simulink library "M160_lib"  (Simulink 7.8)
settings: Solver=FixedStepDiscrete  StartTime=0.0  StopTime=10.0  RelTol=1e-3
PreLoadFcn:
  | update_path
undefined symbols (not defined in the file): Afr_atCool2facLambdaReqCorr_CUR_x, Afr_atCool2facLambdaReqCorr_CUR_y, Afr_atMani2facLambdaReqCorr_CUR_x, Afr_atMani2facLambdaReqCorr_CUR_y, Afr_facLambdaReqMan, Afr_facRatioMan, Afr_facStoich, Afr_flgLambdaReqOverride, Afr_flgRatioOverride, Afr_rpmEngSpdfacRelAir2facLambdaReqBase_MAP_x, Afr_rpmEngSpdfacRelAir2facLambdaReqBase_MAP_y, Afr_rpmEngSpdfacRelAir2facLambdaReqBase_MAP_z, Ais_flgAirInjReacPumpOverride, Ais_stAirInjReacPumpMan, Amc_flgAirMassFlowOverride, Amc_uSens2AirMassFlow_CUR_x, Amc_uSens2AirMassFlow_CUR_y, Amc_uSensMaxValid, Amc_uSensMinValid, Amf_facRelAirMan, Amf_flgAirMassPerStrOverride, Amf_flgRelAirOverride, Amf_flgSwitch2AirMassFlowMeter, Amf_mAirPerStrMan, Amf_pManiEngSpd2facRelAirCorr_MAP_x, Amf_pManiEngSpd2facRelAirCorr_MAP_y, Amf_pManiEngSpd2facRelAirCorr_MAP_z, Amf_rpmEngSpd2facTempCorr_CUR_x, Amf_rpmEngSpd2facTempCorr_CUR_y, Amf_shcSpecGasConst_C, Amf_volEngDisp_C, Apv_facAirPumpRateMan, Apv_factor, Apv_flgAirPumpRateOverride, Apv_tiPeriod_C, Bvc_rVoltDivHigh, Bvc_rVoltDivLow, Bvc_uBattMax, Bvc_uBattMin, CDRV_E_OK_, Cov_facChOverVlvRateMan, Cov_factor, Cov_flgChOverVlvRateOverride, Cov_tiPeriod_C, Cpc_atManiTmp2facPresCorr_CUR_x, Cpc_atManiTmp2facPresCorr_CUR_y, Cpc_flgPChargeOverride, Cpc_uSens2pManiBase_CUR_x, Cpc_uSens2pManiBase_CUR_y, Ctc_rPullUp_C, Ctc_rSens2atCool_CUR_x, Ctc_rSens2atCool_CUR_y, Ctc_uSensMaxValid, Ctc_uSensMinValid, Ctc_uSupply, Doh_OutputDiagnosisOverride, dummy_facAirPumpRateReq, dummy_facChOverVlvRateReq, dummy_flgInterCoolerOverride, dummy_flgKl50Override ... (+243)
libraries: simulink x36, ehooks_lib x3
(part 7 of 8)

== system M160_lib/Sensors/Egc/G1_ADC_Input_Receive ==
  Data Type Conversion : DataTypeConversion  OutMin=0.0  OutMax=5.0  OutDataTypeStr=single
  Data Type Conversion1 : DataTypeConversion  OutMin=0.0  OutMax=1.0  OutDataTypeStr=boolean
  FlexECU_DevLib_FcnAPI_Wrapper_SFcn : S-Function  FunctionName=ehooks_medc17flex_devlib_basic_io_fcncall  Parameters=NoInputPorts, NoOutputPorts, InputPortDataTypes, OutputPortDataTypes, CFunctionArgTypes, CFunctionName, ChannelName  EnableBusSupport=off  mask{NoInputPorts=0, NoOutputPorts=2, InputPortDataTypes=, OutputPortDataTypes=uint8,int16, CFunctionArgTypes=ret,ref, CFunctionName=DevLib_Adc_Get, ChannelName=I_A_AN08}
      mask prompts: NoInputPorts "Number of input ports"; NoOutputPorts "Number of output ports"; InputPortDataTypes "Input port data types"; OutputPortDataTypes "Output port data types"; CFunctionArgTypes "C function argument types"; CFunctionName "C function name"; ChannelName "Channel (pin) name"
      mask Display: disp('EHOOKS FlexECU\nDevLib Wrapper\nS-Function')
  Gain : Gain  Gain=5/1023  OutDataTypeStr=Inherit: Same as input
  status : Outport
  uRaw : Outport  Port=2
  wires:
  Data Type Conversion1/1 -> status/1
  Data Type Conversion/1 -> Gain/1
  FlexECU_DevLib_FcnAPI_Wrapper_SFcn/2 -> Data Type Conversion/1
  FlexECU_DevLib_FcnAPI_Wrapper_SFcn/1 -> Data Type Conversion1/1
  Gain/1 -> uRaw/1

== system M160_lib/Sensors/Egc/G1_ADC_Input_Receive1 ==
  Data Type Conversion : DataTypeConversion  OutMin=0.0  OutMax=5.0  OutDataTypeStr=single
  Data Type Conversion1 : DataTypeConversion  OutMin=0.0  OutMax=1.0  OutDataTypeStr=boolean
  FlexECU_DevLib_FcnAPI_Wrapper_SFcn : S-Function  FunctionName=ehooks_medc17flex_devlib_basic_io_fcncall  Parameters=NoInputPorts, NoOutputPorts, InputPortDataTypes, OutputPortDataTypes, CFunctionArgTypes, CFunctionName, ChannelName  EnableBusSupport=off  mask{NoInputPorts=0, NoOutputPorts=2, InputPortDataTypes=, OutputPortDataTypes=uint8,int16, CFunctionArgTypes=ret,ref, CFunctionName=DevLib_Adc_Get, ChannelName=I_A_AN13}
      mask prompts: NoInputPorts "Number of input ports"; NoOutputPorts "Number of output ports"; InputPortDataTypes "Input port data types"; OutputPortDataTypes "Output port data types"; CFunctionArgTypes "C function argument types"; CFunctionName "C function name"; ChannelName "Channel (pin) name"
      mask Display: disp('EHOOKS FlexECU\nDevLib Wrapper\nS-Function')
  Gain : Gain  Gain=5/1023  OutDataTypeStr=Inherit: Same as input
  status : Outport
  uRaw : Outport  Port=2
  wires:
  Data Type Conversion1/1 -> status/1
  Data Type Conversion/1 -> Gain/1
  FlexECU_DevLib_FcnAPI_Wrapper_SFcn/2 -> Data Type Conversion/1
  FlexECU_DevLib_FcnAPI_Wrapper_SFcn/1 -> Data Type Conversion1/1
  Gain/1 -> uRaw/1

== system M160_lib/Sensors/Egc/LowpassT ==
  initValue : Inport
  Ta : Inport  Port=2
  T : Inport  Port=3
  in : Inport  Port=4
  Add2 : Sum  OutDataTypeStr=Inherit: Same as first input
  Divide1 : Product  Inputs=*/  OutDataTypeStr=Inherit: Same as first input
  MATLAB Function : MATLAB Function  TreatAsAtomicUnit=on
  Product1 : Product  OutDataTypeStr=Inherit: Same as first input
  Product2 : Product  OutDataTypeStr=single
  Subtract1 : Sum  Inputs=+-
  Switch1 : Switch  Threshold=1
  Unit Delay4 : UnitDelay  SampleTime=-1
  Unit Delay5 : UnitDelay  SampleTime=-1
  Unit Delay6 : UnitDelay  SampleTime=-1
  Out : Outport
  wires:
  initValue/1 -> Switch1/3
  Switch1/1 -> Out/1
  MATLAB Function/1(x) -> Divide1/2
  MATLAB Function/2(y) -> Switch1/2, Product2/1
  Ta/1 -> Divide1/1
  T/1 -> MATLAB Function/1(u)
  Divide1/1 -> Unit Delay6/1
  Subtract1/1 -> Product1/2
  Product1/1 -> Add2/1
  Unit Delay5/1 -> Add2/2
  Unit Delay6/1 -> Product1/1
  Unit Delay4/1 -> Subtract1/2
  in/1 -> Subtract1/1
  Product2/1 -> Switch1/1, Unit Delay4/1, Unit Delay5/1
  Add2/1 -> Product2/2

== system M160_lib/Sensors/Egc/LowpassT_Fcn ==
  initValue : Inport
  In : Inport  Port=2
  T : Inport  Port=3
  Discrete Transfer Fcn : DiscreteTransferFcn  Denominator=[Egc_tiTEgasFilt/0.01 1-Egc_tiTEgasFilt/0.01]  SampleTime=-1  OutDataTypeStr=Inherit: Same as input
  MATLAB Function : MATLAB Function  TreatAsAtomicUnit=on
  Product1 : Product  OutDataTypeStr=single
  Switch1 : Switch  Threshold=1
  Out : Outport
  wires:
  MATLAB Function/1(y) -> Switch1/2, Product1/1
  T/1 -> MATLAB Function/1(u)
  initValue/1 -> Switch1/3
  Switch1/1 -> Out/1
  Product1/1 -> Switch1/1
  Discrete Transfer Fcn/1 -> Product1/2
  In/1 -> Discrete Transfer Fcn/1

== system M160_lib/Sensors/Klemme50/G1_Digital_Input_Receive ==
  Data Type Conversion2 : DataTypeConversion  OutMin=0.0  OutMax=1.0  OutDataTypeStr=boolean
  Data Type Conversion3 : DataTypeConversion  OutMin=0.0  OutMax=1.0  OutDataTypeStr=boolean
  FlexECU_DevLib_FcnAPI_Wrapper_SFcn : S-Function  FunctionName=ehooks_medc17flex_devlib_basic_io_fcncall  Parameters=NoInputPorts, NoOutputPorts, InputPortDataTypes, OutputPortDataTypes, CFunctionArgTypes, CFunctionName, ChannelName  EnableBusSupport=off  mask{NoInputPorts=0, NoOutputPorts=2, InputPortDataTypes=, OutputPortDataTypes=uint8,uint8, CFunctionArgTypes=ret,ref, CFunctionName=DevLib_Dio_Get, ChannelName=I_S_DIG17}
      mask prompts: NoInputPorts "Number of input ports"; NoOutputPorts "Number of output ports"; InputPortDataTypes "Input port data types"; OutputPortDataTypes "Output port data types"; CFunctionArgTypes "C function argument types"; CFunctionName "C function name"; ChannelName "Channel (pin) name"
      mask Display: disp('EHOOKS FlexECU\nDevLib Wrapper\nS-Function')
  status : Outport
  stRaw1 : Outport  Port=2
  wires:
  FlexECU_DevLib_FcnAPI_Wrapper_SFcn/2 -> Data Type Conversion2/1
  FlexECU_DevLib_FcnAPI_Wrapper_SFcn/1 -> Data Type Conversion3/1
  Data Type Conversion3/1 -> status/1
  Data Type Conversion2/1 -> stRaw1/1

== system M160_lib/Sensors/Mpc/Mpc_calc ==
  Epm_rpmEngSpd : Inport
  Mpc_pMani : Inport  Port=2
  Mpc_flgError : Inport  Port=3
  function : TriggerPort  TriggerType=function-call
  Accumulator : Subsystem
      mask Description: Accumulator
      mask Display: image(imread('Accumulator.jpg'))
  Constant1 : Constant  Value=0  OutDataTypeStr=single
  Constant2 : Constant  Value=0  OutDataTypeStr=single
  Constant6 : Constant  Value=30  OutDataTypeStr=single
  Counter : Subsystem
      mask Description: Counter
      mask Display: image(imread('Counter.jpg'))
  Divide : Product  Inputs=*/  OutDataTypeStr=single
  Logical Operator2 : Logic  Operator=NOT  AllPortsSameDT=off  OutDataTypeStr=boolean
  Logical Operator3 : Logic  AllPortsSameDT=off  OutDataTypeStr=boolean
  Relational Operator : RelationalOperator  Operator=>  OutDataTypeStr=boolean
  Relational Operator1 : RelationalOperator  Operator=>  OutDataTypeStr=boolean
  Switch : Switch  Threshold=1
  Switch1 : Switch  Threshold=1
  Mpc_pManiFilt : Outport
  wires:
  Switch1/1 -> Counter/1(in), Accumulator/1(in)
  Logical Operator3/1 -> Switch1/2
  Divide/1 -> Switch/1
  Switch/1 -> Mpc_pManiFilt/1  "Mpc_pManiFilt"
  Accumulator/1(Out2) -> Divide/1  "Mpc_pAccu"
  Constant2/1 -> Switch1/3, Accumulator/2(initValue)
  Relational Operator1/1 -> Switch/2
  Constant1/1 -> Relational Operator1/2
  Counter/1(Out1) -> Relational Operator1/1, Divide/2  "Mpc_nrValues"
  Constant6/1 -> Relational Operator/2
  Epm_rpmEngSpd/1 -> Relational Operator/1
  Relational Operator/1 -> Logical Operator3/1
  Logical Operator2/1 -> Logical Operator3/2
  Mpc_pMani/1 -> Switch/3, Switch1/1
  Mpc_flgError/1 -> Logical Operator2/1

== system M160_lib/Sensors/Mpc/Mpc_get ==
  Mtc_atMani : Inport
  function : TriggerPort  TriggerType=function-call
  G1_ADC_Input_Receive : Subsystem  LoadFcn=ehooks_medc17flex_devlib_io_block('load');  InitFcn=ehooks_medc17flex_devlib_io_block('init');  StartFcn=ehooks_medc17flex_devlib_io_block('start');  StopFcn=ehooks_medc17flex_devlib_io_block('stop');  ClipboardFcn=ehooks_medc17flex_devlib_io_block('clipboard', 0); % Second argument just needed to indicate null block. See callback handler.  mask{ChannelName=I_A_AN05}
      mask prompts: ChannelName "Channel name"
      mask init:
      | ehooks_medc17flex_devlib_io_block('mask_init');
      settings: AttributesFormatString=Channel name: '%<ChannelName>'  CopyFcn=ehooks_medc17flex_devlib_io_block('copy');  DeleteFcn=ehooks_medc17flex_devlib_io_block('delete');  UndoDeleteFcn=ehooks_medc17flex_devlib_io_block('undo_delete');  ModelCloseFcn=ehooks_medc17flex_devlib_io_block('model_close');  PreSaveFcn=ehooks_medc17flex_devlib_io_block('pre_save');  PostSaveFcn=ehooks_medc17flex_devlib_io_block('post_save');  NameChangeFcn=ehooks_medc17flex_devlib_io_block('name_change');  DestroyFcn=ehooks_medc17flex_devlib_io_block('destroy', 0); % Second argument just needed to indicate null block. See callback handler.  OpenFcn=ehooks_medc17flex_devlib_io_block('open');  CloseFcn=ehooks_medc17flex_devlib_io_block('close');  ParentCloseFcn=ehooks_medc17flex_devlib_io_block('parent_close');  MoveFcn=ehooks_medc17flex_devlib_io_block('move');
      mask StyleString: popup(<empty>|I_A_AN01|I_A_AN02|I_A_AN03|I_A_AN05|I_A_AN06|I_A_AN07|I_A_AN08|I_A_AN10|I_A_AN11|I_A_AN12|I_A_AN13|I_A_AN14|I_A_AN15|I_A_AN16|I_A_AN17|I_A_AN18|I_A_AN19|I_A_AN20|I_A_AN21|I_A_AN23|I_A_AN32|I_A_AN35|I_A_AN36|I_A_AN37|I_A_AN39|I_A_AN100|I_A_AN101|I_A_AN103|I_A_AN104|I_A_AN105|I_A_AN106)
      mask Display: image(imread('Input_Analog.jpg'))
  Interval Test : simulink/Logic and Bit Operations/Interval Test  IntervalClosedRight=on  uplimit=Mpc_uSensMaxValid  IntervalClosedLeft=on  lowlimit=Mpc_uSensMinValid  OutDataTypeStr=boolean
  Logical Operator : Logic  Operator=NOT  AllPortsSameDT=off  OutDataTypeStr=boolean
  Logical Operator1 : Logic  Operator=NOT  AllPortsSameDT=off  OutDataTypeStr=boolean
  Logical Operator4 : Logic  Operator=OR  AllPortsSameDT=off  OutDataTypeStr=boolean
  Mpc_atManiTmp2facPresCorr_CUR : Lookup_n-D  NumberOfTableDimensions=1  BreakpointsForDimension1=Mpc_atManiTmp2facPresCorr_CUR_x  BreakpointsForDimension1DataTypeStr=Inherit: Inherit from 'Breakpoint data'  Table=Mpc_atManiTmp2facPresCorr_CUR_y  TableDataTypeStr=Inherit: Inherit from 'Table data'  ExtrapMethod=Clip  OutDataTypeStr=Inherit: Inherit from 'Table data'  InputSameDT=on
  Mpc_uSens2pManiBase_CUR : Lookup_n-D  NumberOfTableDimensions=1  BreakpointsForDimension1=Mpc_uSens2pManiBase_CUR_x  BreakpointsForDimension1DataTypeStr=Inherit: Inherit from 'Breakpoint data'  Table=Mpc_uSens2pManiBase_CUR_y  TableDataTypeStr=Inherit: Inherit from 'Table data'  ExtrapMethod=Clip  OutDataTypeStr=Inherit: Inherit from 'Table data'  InputSameDT=on
  Product : Product  OutDataTypeStr=Inherit: Same as first input
  Mpc_flgError : Outport
  Ctc_atCool1 : Outport  Port=2
  wires:
  Logical Operator4/1 -> Mpc_flgError/1  "Mpc_flgError"
  Logical Operator1/1 -> Logical Operator4/2
  Logical Operator/1 -> Logical Operator4/1
  Interval Test/1 -> Logical Operator1/1
  G1_ADC_Input_Receive/2(uRaw) -> Mpc_uSens2pManiBase_CUR/1, Interval Test/1  "Mpc_uSens"
  G1_ADC_Input_Receive/1(status) -> Logical Operator/1  "Mpc_stIOError"
  Product/1 -> Ctc_atCool1/1  "Mpc_pMani"
  Mtc_atMani/1 -> Mpc_atManiTmp2facPresCorr_CUR/1
  Mpc_uSens2pManiBase_CUR/1 -> Product/1
  Mpc_atManiTmp2facPresCorr_CUR/1 -> Product/2

== system M160_lib/Sensors/Mpc/Mpc_pMani_calc ==
  ECU_FcnCallTrigger_Source_DownStream : Subsystem  TreatAsAtomicUnit=on
  TriggerOut : Outport
  wires:
  ECU_FcnCallTrigger_Source_DownStream/1(TriggerOut) -> TriggerOut/1

== system M160_lib/Sensors/Mpc/Mpc_pMani_get ==
  ECU_FcnCallTrigger_Source_DownStream : Subsystem  TreatAsAtomicUnit=on
  TriggerOut : Outport
  wires:
  ECU_FcnCallTrigger_Source_DownStream/1(TriggerOut) -> TriggerOut/1

== system M160_lib/Sensors/Mtc/G1_ADC_Input_Receive ==
  Data Type Conversion2 : DataTypeConversion  OutMin=0.0  OutMax=5.0  OutDataTypeStr=single
  Data Type Conversion3 : DataTypeConversion  OutMin=0.0  OutMax=1.0  OutDataTypeStr=boolean
  FlexECU_DevLib_FcnAPI_Wrapper_SFcn : S-Function  FunctionName=ehooks_medc17flex_devlib_basic_io_fcncall  Parameters=NoInputPorts, NoOutputPorts, InputPortDataTypes, OutputPortDataTypes, CFunctionArgTypes, CFunctionName, ChannelName  EnableBusSupport=off  mask{NoInputPorts=0, NoOutputPorts=2, InputPortDataTypes=, OutputPortDataTypes=uint8,int16, CFunctionArgTypes=ret,ref, CFunctionName=DevLib_Adc_Get, ChannelName=I_A_AN14}
      mask prompts: NoInputPorts "Number of input ports"; NoOutputPorts "Number of output ports"; InputPortDataTypes "Input port data types"; OutputPortDataTypes "Output port data types"; CFunctionArgTypes "C function argument types"; CFunctionName "C function name"; ChannelName "Channel (pin) name"
      mask Display: disp('EHOOKS FlexECU\nDevLib Wrapper\nS-Function')
  Gain : Gain  Gain=5/1023  OutDataTypeStr=Inherit: Same as input
  status : Outport
  uRaw : Outport  Port=2
  wires:
  FlexECU_DevLib_FcnAPI_Wrapper_SFcn/1 -> Data Type Conversion3/1
  FlexECU_DevLib_FcnAPI_Wrapper_SFcn/2 -> Data Type Conversion2/1
  Gain/1 -> uRaw/1
  Data Type Conversion3/1 -> status/1
  Data Type Conversion2/1 -> Gain/1

== system M160_lib/Sensors/Opc/G1_Digital_Input_Receive ==
  Data Type Conversion2 : DataTypeConversion  OutMin=0.0  OutMax=1.0  OutDataTypeStr=boolean
  Data Type Conversion3 : DataTypeConversion  OutMin=0.0  OutMax=1.0  OutDataTypeStr=boolean
  FlexECU_DevLib_FcnAPI_Wrapper_SFcn : S-Function  FunctionName=ehooks_medc17flex_devlib_basic_io_fcncall  Parameters=NoInputPorts, NoOutputPorts, InputPortDataTypes, OutputPortDataTypes, CFunctionArgTypes, CFunctionName, ChannelName  EnableBusSupport=off  mask{NoInputPorts=0, NoOutputPorts=2, InputPortDataTypes=, OutputPortDataTypes=uint8,uint8, CFunctionArgTypes=ret,ref, CFunctionName=DevLib_Dio_Get, ChannelName=I_S_DIG13}
      mask prompts: NoInputPorts "Number of input ports"; NoOutputPorts "Number of output ports"; InputPortDataTypes "Input port data types"; OutputPortDataTypes "Output port data types"; CFunctionArgTypes "C function argument types"; CFunctionName "C function name"; ChannelName "Channel (pin) name"
      mask Display: disp('EHOOKS FlexECU\nDevLib Wrapper\nS-Function')
  status : Outport
  stRaw1 : Outport  Port=2
  wires:
  FlexECU_DevLib_FcnAPI_Wrapper_SFcn/2 -> Data Type Conversion2/1
  FlexECU_DevLib_FcnAPI_Wrapper_SFcn/1 -> Data Type Conversion3/1
  Data Type Conversion3/1 -> status/1
  Data Type Conversion2/1 -> stRaw1/1

== system M160_lib/Actuators/Ivc/Ivc/G1_InjVlvPFI_SetParam ==
  te_i : Inport
  tez_i1 : Inport  Port=2
  tez_i2 : Inport  Port=3
  tez_i3 : Inport  Port=4
  tez_i4 : Inport  Port=5
  tez_i5 : Inport  Port=6
  tez_i6 : Inport  Port=7
  tez_i7 : Inport  Port=8
  tez_i8 : Inport  Port=9
  dtemnkt_w : Inport  Port=10
  tvub_w : Inport  Port=11
  B_nsp : Inport  Port=12
  B_stendes : Inport  Port=13
  evz_austot : Inport  Port=14
  wea : Inport  Port=15
  weea_1 : Inport  Port=16
  weea_2 : Inport  Port=17
  weea_3 : Inport  Port=18
  weestim : Inport  Port=19
  wes : Inport  Port=20
  DTC_PFI_B_nsp : DataTypeConversion  OutDataTypeStr=uint8  RndMeth=Nearest
  DTC_PFI_B_stendes : DataTypeConversion  OutDataTypeStr=uint8  RndMeth=Nearest
  DTC_PFI_B_weea_1 : DataTypeConversion  OutDataTypeStr=uint8  RndMeth=Nearest
  DTC_PFI_B_weea_2 : DataTypeConversion  OutDataTypeStr=uint8
  DTC_PFI_B_weea_3 : DataTypeConversion  OutDataTypeStr=uint8  RndMeth=Nearest
  DTC_PFI_B_weestsim : DataTypeConversion  OutDataTypeStr=uint8  RndMeth=Nearest
  DTC_PFI_CdrvError : DataTypeConversion  OutDataTypeStr=single
  DTC_PFI_dtemnkt_w : DataTypeConversion  OutDataTypeStr=uint16  RndMeth=Nearest
  DTC_PFI_evz_austot : DataTypeConversion  OutDataTypeStr=uint8  RndMeth=Nearest
  DTC_PFI_te_l : DataTypeConversion  OutDataTypeStr=uint32  RndMeth=Nearest
  DTC_PFI_tez_8 : DataTypeConversion  OutDataTypeStr=uint32  RndMeth=Nearest
  DTC_PFI_tez_i{1..7} (7 alike) : DataTypeConversion  OutDataTypeStr=uint32  RndMeth=Nearest
  DTC_PFI_tvub_w : DataTypeConversion  OutDataTypeStr=uint16  RndMeth=Nearest
  DTC_PFI_wea : DataTypeConversion  OutDataTypeStr=uint8  RndMeth=Nearest
  DTC_PFI_wes : DataTypeConversion  OutDataTypeStr=uint8  RndMeth=Nearest
  FlexECU_SFcn_PFI_inj : S-Function  FunctionName=ehooks_medc17flex_devlib_ign_struct_fcncall  Parameters=NoInputPorts, NoOutputPorts, InputPortDataTypes, OutputPortDataTypes, CFunctionArgTypes, CFunctionName, StructMemberNames, StructTypeName, InputPortDataWidths, OutputPortDataWidths  EnableBusSupport=off  mask{NoInputPorts=11, NoOutputPorts=1, InputPortDataTypes=uint32, uint32, uint16, uint16,uint8,uint8,uint8,uint8,uint8,uint8,uint8, OutputPortDataTypes=uint8, CFunctionArgTypes=ret,val, refin, val,val,val,val,val, val, refin, val, val, CFunctionName=InjVlvPfi_SetParam, StructMemberNames=te_l,  tez_l, dtemnkt_w, tvub_w, B_nsp, B_stendes, evz_austot, wea, weea, weestsim, wes, StructTypeName=InjVlvPfiInterface_type, InputPortDataWidths=1,8,1,1,1,1,1,1,3,1,1, OutputPortDataWidths=1}
      mask prompts: NoInputPorts "Number of input ports"; NoOutputPorts "Number of output ports"; InputPortDataTypes "Input port data types"; OutputPortDataTypes "Output port data types"; CFunctionArgTypes "C function argument types"; CFunctionName "C function name"; StructMemberNames "Structure member names"; StructTypeName "Structure type name"; InputPortDataWidths "Input port widths"; OutputPortDataWidths "Output port widths"
      mask Display: disp('EHOOKS FlexECU\nDevLib Wrapper\nS-Function')
  Mux : Mux  Inputs=8
  Mux1 : Mux  Inputs=3
  Cdrv_Error : Outport
  wires:
  DTC_PFI_CdrvError/1 -> Cdrv_Error/1
  FlexECU_SFcn_PFI_inj/1 -> DTC_PFI_CdrvError/1
  DTC_PFI_B_stendes/1 -> FlexECU_SFcn_PFI_inj/6
  B_stendes/1 -> DTC_PFI_B_stendes/1
  DTC_PFI_B_nsp/1 -> FlexECU_SFcn_PFI_inj/5
  B_nsp/1 -> DTC_PFI_B_nsp/1
  DTC_PFI_tvub_w/1 -> FlexECU_SFcn_PFI_inj/4
  tvub_w/1 -> DTC_PFI_tvub_w/1
  DTC_PFI_dtemnkt_w/1 -> FlexECU_SFcn_PFI_inj/3
  dtemnkt_w/1 -> DTC_PFI_dtemnkt_w/1
  te_i/1 -> DTC_PFI_te_l/1
  DTC_PFI_evz_austot/1 -> FlexECU_SFcn_PFI_inj/7
  DTC_PFI_wea/1 -> FlexECU_SFcn_PFI_inj/8
  DTC_PFI_B_weestsim/1 -> FlexECU_SFcn_PFI_inj/10
  DTC_PFI_wes/1 -> FlexECU_SFcn_PFI_inj/11
  evz_austot/1 -> DTC_PFI_evz_austot/1
  wea/1 -> DTC_PFI_wea/1
  weea_1/1 -> DTC_PFI_B_weea_1/1
  weestim/1 -> DTC_PFI_B_weestsim/1
  wes/1 -> DTC_PFI_wes/1
  DTC_PFI_te_l/1 -> FlexECU_SFcn_PFI_inj/1
  tez_i1/1 -> DTC_PFI_tez_i1/1
  tez_i2/1 -> DTC_PFI_tez_i2/1
  tez_i3/1 -> DTC_PFI_tez_i3/1
  tez_i4/1 -> DTC_PFI_tez_i4/1
  tez_i5/1 -> DTC_PFI_tez_i5/1
  tez_i6/1 -> DTC_PFI_tez_i6/1
  tez_i7/1 -> DTC_PFI_tez_i7/1
  tez_i8/1 -> DTC_PFI_tez_8/1
  DTC_PFI_tez_i1/1 -> Mux/1
  DTC_PFI_tez_i2/1 -> Mux/2
  DTC_PFI_tez_i3/1 -> Mux/3
  DTC_PFI_tez_i4/1 -> Mux/4
  DTC_PFI_tez_i5/1 -> Mux/5
  DTC_PFI_tez_i6/1 -> Mux/6
  DTC_PFI_tez_i7/1 -> Mux/7
  DTC_PFI_tez_8/1 -> Mux/8
  Mux/1 -> FlexECU_SFcn_PFI_inj/2  "tez_xxx"
  weea_2/1 -> DTC_PFI_B_weea_2/1
  weea_3/1 -> DTC_PFI_B_weea_3/1
  DTC_PFI_B_weea_1/1 -> Mux1/1
  DTC_PFI_B_weea_2/1 -> Mux1/2
  DTC_PFI_B_weea_3/1 -> Mux1/3
  Mux1/1 -> FlexECU_SFcn_PFI_inj/9  "weea_xxx"

== system M160_lib/Actuators/Ivc/Ivc_Diag/G1_Inj_Set_DEVE_forPFI ==
  B_desee : Inport
  B_sa : Inport  Port=2
  DTC_PFI_DEVE_Bdesee : DataTypeConversion  OutDataTypeStr=uint8  RndMeth=Nearest
  DTC_PFI_DEVE_Bsa : DataTypeConversion  OutDataTypeStr=uint8  RndMeth=Nearest
  DTC_PFI_DEVE_Bsa1 : DataTypeConversion  OutDataTypeStr=single
  FlexECU_SFcn_PFI_inj : S-Function  FunctionName=ehooks_medc17flex_devlib_ign_struct_fcncall  Parameters=NoInputPorts, NoOutputPorts, InputPortDataTypes, OutputPortDataTypes, CFunctionArgTypes, CFunctionName, StructMemberNames, StructTypeName, InputPortDataWidths, OutputPortDataWidths  EnableBusSupport=off  mask{NoInputPorts=2, NoOutputPorts=1, InputPortDataTypes=uint8,uint8, OutputPortDataTypes=uint8, CFunctionArgTypes=ret, val, val, CFunctionName=InjVlvDeve_SetParam, StructMemberNames=B_desee, B_sa, StructTypeName=InjVlvDeveInterface_type, InputPortDataWidths=1,1, OutputPortDataWidths=1}
      mask prompts: NoInputPorts "Number of input ports"; NoOutputPorts "Number of output ports"; InputPortDataTypes "Input port data types"; OutputPortDataTypes "Output port data types"; CFunctionArgTypes "C function argument types"; CFunctionName "C function name"; StructMemberNames "Structure member names"; StructTypeName "Structure type name"; InputPortDataWidths "Input port widths"; OutputPortDataWidths "Output port widths"
      mask Display: disp('EHOOKS FlexECU\nDevLib Wrapper\nS-Function')
  Cdrv_Error : Outport
  wires:
  DTC_PFI_DEVE_Bsa/1 -> FlexECU_SFcn_PFI_inj/2
  B_sa/1 -> DTC_PFI_DEVE_Bsa/1
  B_desee/1 -> DTC_PFI_DEVE_Bdesee/1
  DTC_PFI_DEVE_Bdesee/1 -> FlexECU_SFcn_PFI_inj/1
  FlexECU_SFcn_PFI_inj/1 -> DTC_PFI_DEVE_Bsa1/1
  DTC_PFI_DEVE_Bsa1/1 -> Cdrv_Error/1

== system M160_lib/Actuators/Tvc/ThrottleValveControl/PID_Limit_AWU ==
  Tn : Inport
  Tv : Inport  Port=2
  Ta : Inport  Port=3
  Kp : Inport  Port=4
  in : Inport  Port=5
  initValue : Inport  Port=6
  outMax : Inport  Port=7
  outMin : Inport  Port=8
  Add : Sum  OutDataTypeStr=Inherit: Same as first input
  Add1 : Sum  Inputs=+++  OutDataTypeStr=Inherit: Same as first input
  Constant1 : Constant  Value=0.0  OutDataTypeStr=single
  Constant10 : Constant  Value=0.0  OutDataTypeStr=single
  Divide : Product  Inputs=*/  OutDataTypeStr=Inherit: Same as first input
  Divide1 : Product  Inputs=*/  OutDataTypeStr=Inherit: Same as first input
  Interval Test : simulink/Logic and Bit Operations/Interval Test  IntervalClosedRight=on  uplimit=Tvc_facDutycyclePIDLimitMax  IntervalClosedLeft=on  lowlimit=Tvc_facDutycyclePIDLimitMin  OutDataTypeStr=boolean
  Limiter : Subsystem
      mask Description: Limiter
      mask Display: image(imread('Limiter.jpg'))
  Product : Product  OutDataTypeStr=Inherit: Same as first input
  Product1 : Product  OutDataTypeStr=Inherit: Same as first input
  Product2 : Product  Inputs=3  OutDataTypeStr=Inherit: Same as first input
  Product3 : Product  OutDataTypeStr=Inherit: Same as first input
  Subtract : Sum  Inputs=+-  OutDataTypeStr=Inherit: Same as first input
  Switch1 : Switch  Threshold=1
  Switch2 : Switch  Threshold=1
  Unit Delay1 : UnitDelay  SampleTime=-1
  Unit Delay2 : UnitDelay  SampleTime=-1
  Tvc_facDutycycleCorr : Outport
  wires:
  Constant10/1 -> Switch2/3
  Product2/1 -> Switch2/1
  Interval Test/1 -> Switch2/2
  Unit Delay2/1 -> Add/2, Add1/2
  Add/1 -> Unit Delay2/1
  Unit Delay1/1 -> Subtract/2
  Kp/1 -> Product/1, Product3/2, Divide1/1
  Tv/1 -> Product/2
  Product/1 -> Divide/1
  Ta/1 -> Product2/1, Divide/2
  Divide/1 -> Product1/1
  Tn/1 -> Divide1/2
  in/1 -> Product2/2, Product3/1, Subtract/1, Unit Delay1/1  "inOLD"
  Divide1/1 -> Product2/3
  Subtract/1 -> Product1/2
  Switch2/1 -> Add/1
  Product3/1 -> Add1/3
  Product1/1 -> Add1/1
  Add1/1 -> Limiter/2(in), Interval Test/1
  outMin/1 -> Limiter/3(min)
  outMax/1 -> Limiter/1(max)
  Constant1/1 -> Switch1/3
  initValue/1 -> Switch1/2
  Switch1/1 -> Tvc_facDutycycleCorr/1
  Limiter/1(return) -> Switch1/1

== system M160_lib/Actuators/Tvc/ThrottleValveControl/PID_Limit_AWU_Fcn ==
  in : Inport
  initValue : Inport  Port=2
  Constant1 : Constant  Value=0.0  OutDataTypeStr=single
  Discrete PID Controller : simulink/Continuous/PID Controller  Controller=PID  TimeDomain=Discrete-time  SampleTime=-1  IntegratorMethod=Forward Euler  FilterMethod=Forward Euler  Form=Parallel  P=Tvc_facKDutycycle  I=Tvc_facKDutycycle/Tvc_tiTnDutycycle  D=Tvc_facKDutycycle*Tvc_tiTvDutycycle  N=Tvc_facKDutycycle*Tvc_tiTvDutycycle/0.01  InitialConditionSource=internal  InitialConditionForIntegrator=0  InitialConditionForFilter=0  ExternalReset=none  LimitOutput=on  UpperSaturationLimit=Tvc_facDutycyclePIDLimitMax  LowerSaturationLimit=Tvc_facDutycyclePIDLimitMin  LinearizeAsGain=off  AntiWindupMode=none  Kb=1  TrackingMode=off  Kt=1  PParamMin=[]  PParamMax=[]  IParamMin=[]  IParamMax=[]  DParamMin=[]  DParamMax=[]  NParamMin=[]  NParamMax=[]  KbParamMin=[]  KbParamMax=[]  KtParamMin=[]  KtParamMax=[]  POutMin=[]  POutMax=[]  IOutMin=[]  IOutMax=[]  DOutMin=[]  DOutMax=[]  NOutMin=[]  NOutMax=[]  KbOutMin=[]  KbOutMax=[]  KtOutMin=[]  KtOutMax=[]  IntegratorOutMin=[]  IntegratorOutMax=[]  FilterOutMin=[]  FilterOutMax=[]  SumOutMin=[]  SumOutMax=[]  SumI1OutMin=[]  SumI1OutMax=[]  SumI2OutMin=[]  SumI2OutMax=[]  SumI3OutMin=[]  SumI3OutMax=[]  SumDOutMin=[]  SumDOutMax=[]  SaturationOutMin=[]  SaturationOutMax=[]  IntegratorContinuousStateAttributes=''  IntegratorStateMustResolveToSignalObject=off  IntegratorRTWStateStorageClass=Auto  FilterContinuousStateAttributes=''  FilterStateMustResolveToSignalObject=off  FilterRTWStateStorageClass=Auto
  Switch1 : Switch  Threshold=1
  Tvc_facDutycycleCorr : Outport
  wires:
  Switch1/1 -> Tvc_facDutycycleCorr/1
  initValue/1 -> Switch1/2
  Constant1/1 -> Switch1/3
  in/1 -> Discrete PID Controller/1  "inOLD"
  Discrete PID Controller/1 -> Switch1/1

== system M160_lib/Actuators/Tvc/ThrottleValveOutput/G1_HbridgeOut_Ctrl ==
  dutycycle : Inport
  disable : Inport  Port=2
  period : Inport  Port=3
  level : Inport  Port=4
  DTC_HB_Disable : DataTypeConversion  OutDataTypeStr=uint8  RndMeth=Nearest
  DTC_HB_DutyCycle : DataTypeConversion  OutDataTypeStr=int16  RndMeth=Nearest
  DTC_HB_ErrorInfo : DataTypeConversion  OutMin=0.0  OutMax=1.0  OutDataTypeStr=boolean
  DTC_HB_Level : DataTypeConversion  OutDataTypeStr=uint8  RndMeth=Nearest
  DTC_HB_Period : DataTypeConversion  OutDataTypeStr=int16  RndMeth=Nearest
  FlexECU_DevLib_FcnAPI_Wrapper_SFcn : S-Function  FunctionName=ehooks_medc17flex_devlib_basic_io_fcncall  Parameters=NoInputPorts, NoOutputPorts, InputPortDataTypes, OutputPortDataTypes, CFunctionArgTypes, CFunctionName, ChannelName  EnableBusSupport=off  mask{NoInputPorts=4, NoOutputPorts=1, InputPortDataTypes=int16,uint8,int16,uint8, OutputPortDataTypes=uint8, CFunctionArgTypes=ret,val,val,val, val, CFunctionName=DevLib_HBridge_Out, ChannelName=O_T_DC1}
      mask prompts: NoInputPorts "Number of input ports"; NoOutputPorts "Number of output ports"; InputPortDataTypes "Input port data types"; OutputPortDataTypes "Output port data types"; CFunctionArgTypes "C function argument types"; CFunctionName "C function name"; ChannelName "Channel (pin) name"
      mask Display: disp('EHOOKS FlexECU\nDevLib Wrapper\nS-Function')
  Gain : Gain  Gain=100
  status : Outport
  wires:
  Gain/1 -> DTC_HB_DutyCycle/1
  disable/1 -> DTC_HB_Disable/1
  DTC_HB_Disable/1 -> FlexECU_DevLib_FcnAPI_Wrapper_SFcn/2
  DTC_HB_Level/1 -> FlexECU_DevLib_FcnAPI_Wrapper_SFcn/4
  DTC_HB_Period/1 -> FlexECU_DevLib_FcnAPI_Wrapper_SFcn/3
  DTC_HB_ErrorInfo/1 -> status/1
  DTC_HB_DutyCycle/1 -> FlexECU_DevLib_FcnAPI_Wrapper_SFcn/1
  level/1 -> DTC_HB_Level/1
  period/1 -> DTC_HB_Period/1
  FlexECU_DevLib_FcnAPI_Wrapper_SFcn/1 -> DTC_HB_ErrorInfo/1
  dutycycle/1 -> Gain/1

== system M160_lib/Actuators/Tvc/ThrottleValveOutput/G1_Hbridge_Get_error ==
  DTC_HB_GetError : DataTypeConversion  OutMin=0  OutMax=7  OutDataTypeStr=single
  FlexECU_DevLib_FcnAPI_Wrapper_SFcn : S-Function  FunctionName=ehooks_medc17flex_devlib_basic_io_fcncall  Parameters=NoInputPorts, NoOutputPorts, InputPortDataTypes, OutputPortDataTypes, CFunctionArgTypes, CFunctionName, ChannelName  EnableBusSupport=off  mask{NoInputPorts=0, NoOutputPorts=1, InputPortDataTypes=, OutputPortDataTypes=uint8, CFunctionArgTypes=ret, CFunctionName=DevLib_HBridge_GetError, ChannelName=O_T_DC1}
      mask prompts: NoInputPorts "Number of input ports"; NoOutputPorts "Number of output ports"; InputPortDataTypes "Input port data types"; OutputPortDataTypes "Output port data types"; CFunctionArgTypes "C function argument types"; CFunctionName "C function name"; ChannelName "Channel (pin) name"
      mask Display: disp('EHOOKS FlexECU\nDevLib Wrapper\nS-Function')
  status : Outport
  wires:
  FlexECU_DevLib_FcnAPI_Wrapper_SFcn/1 -> DTC_HB_GetError/1
  DTC_HB_GetError/1 -> status/1

== system M160_lib/Actuators/Tvc/ThrottleValvePosition/G1_ADC_Input_Receive ==
  Data Type Conversion : DataTypeConversion  OutMin=0.0  OutMax=5.0  OutDataTypeStr=single
  Data Type Conversion1 : DataTypeConversion  OutMin=0.0  OutMax=1.0  OutDataTypeStr=boolean
  FlexECU_DevLib_FcnAPI_Wrapper_SFcn : S-Function  FunctionName=ehooks_medc17flex_devlib_basic_io_fcncall  Parameters=NoInputPorts, NoOutputPorts, InputPortDataTypes, OutputPortDataTypes, CFunctionArgTypes, CFunctionName, ChannelName  EnableBusSupport=off  mask{NoInputPorts=0, NoOutputPorts=2, InputPortDataTypes=, OutputPortDataTypes=uint8,int16, CFunctionArgTypes=ret,ref, CFunctionName=DevLib_Adc_Get, ChannelName=I_A_AN01}
      mask prompts: NoInputPorts "Number of input ports"; NoOutputPorts "Number of output ports"; InputPortDataTypes "Input port data types"; OutputPortDataTypes "Output port data types"; CFunctionArgTypes "C function argument types"; CFunctionName "C function name"; ChannelName "Channel (pin) name"
      mask Display: disp('EHOOKS FlexECU\nDevLib Wrapper\nS-Function')
  Gain : Gain  Gain=5/1023  OutDataTypeStr=Inherit: Same as input
  status : Outport
  uRaw : Outport  Port=2
  wires:
  Data Type Conversion1/1 -> status/1
  Data Type Conversion/1 -> Gain/1
  FlexECU_DevLib_FcnAPI_Wrapper_SFcn/2 -> Data Type Conversion/1
  FlexECU_DevLib_FcnAPI_Wrapper_SFcn/1 -> Data Type Conversion1/1
  Gain/1 -> uRaw/1

== system M160_lib/Actuators/Tvc/ThrottleValvePosition/G1_ADC_Input_Receive1 ==
  Data Type Conversion : DataTypeConversion  OutMin=0.0  OutMax=5.0  OutDataTypeStr=single
  Data Type Conversion1 : DataTypeConversion  OutMin=0.0  OutMax=1.0  OutDataTypeStr=boolean
  FlexECU_DevLib_FcnAPI_Wrapper_SFcn : S-Function  FunctionName=ehooks_medc17flex_devlib_basic_io_fcncall  Parameters=NoInputPorts, NoOutputPorts, InputPortDataTypes, OutputPortDataTypes, CFunctionArgTypes, CFunctionName, ChannelName  EnableBusSupport=off  mask{NoInputPorts=0, NoOutputPorts=2, InputPortDataTypes=, OutputPortDataTypes=uint8,int16, CFunctionArgTypes=ret,ref, CFunctionName=DevLib_Adc_Get, ChannelName=I_A_AN02}
      mask prompts: NoInputPorts "Number of input ports"; NoOutputPorts "Number of output ports"; InputPortDataTypes "Input port data types"; OutputPortDataTypes "Output port data types"; CFunctionArgTypes "C function argument types"; CFunctionName "C function name"; ChannelName "Channel (pin) name"
      mask Display: disp('EHOOKS FlexECU\nDevLib Wrapper\nS-Function')
  Gain : Gain  Gain=5/1023  OutDataTypeStr=Inherit: Same as input
  status : Outport
  uRaw : Outport  Port=2
  wires:
  Data Type Conversion1/1 -> status/1
  Data Type Conversion/1 -> Gain/1
  FlexECU_DevLib_FcnAPI_Wrapper_SFcn/2 -> Data Type Conversion/1
  FlexECU_DevLib_FcnAPI_Wrapper_SFcn/1 -> Data Type Conversion1/1
  Gain/1 -> uRaw/1

== system M160_lib/Functions/Lcc/PID-Controller/PID_Limit_AWU ==
  Tn : Inport
  Tv : Inport  Port=2
  Ta : Inport  Port=3
  Kp : Inport  Port=4
  in : Inport  Port=5
  initValue : Inport  Port=6
  outMax : Inport  Port=7
  outMin : Inport  Port=8
  Add : Sum  OutDataTypeStr=Inherit: Same as first input
  Add1 : Sum  Inputs=+++  OutDataTypeStr=Inherit: Same as first input
  Constant1 : Constant  Value=Lcc_StartValuePID
  Constant10 : Constant  Value=0.0  OutDataTypeStr=single
  Divide : Product  Inputs=*/  OutDataTypeStr=Inherit: Same as first input
  Divide1 : Product  Inputs=*/  OutDataTypeStr=Inherit: Same as first input
  Interval Test : simulink/Logic and Bit Operations/Interval Test  IntervalClosedRight=on  uplimit=Lcc_LambdaCorrMaxPID  IntervalClosedLeft=on  lowlimit=Lcc_LambdaCorrMinPID  OutDataTypeStr=boolean
  Limiter : Subsystem
      mask Description: Limiter
      mask Display: image(imread('Limiter.jpg'))
  Product : Product  OutDataTypeStr=Inherit: Same as first input
  Product1 : Product  OutDataTypeStr=Inherit: Same as first input
  Product2 : Product  Inputs=3  OutDataTypeStr=Inherit: Same as first input
  Product3 : Product  OutDataTypeStr=Inherit: Same as first input
  Subtract : Sum  Inputs=+-  OutDataTypeStr=Inherit: Same as first input
  Switch1 : Switch  Threshold=1
  Switch2 : Switch  Threshold=1
  Unit Delay1 : UnitDelay  SampleTime=-1
  Unit Delay2 : UnitDelay  SampleTime=-1
  Lcc_facLambdaPIDController : Outport
  wires:
  Constant10/1 -> Switch2/3
  Product2/1 -> Switch2/1
  Interval Test/1 -> Switch2/2
  Unit Delay2/1 -> Add/2, Add1/2
  Add/1 -> Unit Delay2/1
  Unit Delay1/1 -> Subtract/2
  Kp/1 -> Product/1, Product3/2, Divide1/1
  Tv/1 -> Product/2
  Product/1 -> Divide/1
  Ta/1 -> Product2/1, Divide/2
  Divide/1 -> Product1/1
  Tn/1 -> Divide1/2
  in/1 -> Product2/2, Product3/1, Subtract/1, Unit Delay1/1  "inOLD"
  Divide1/1 -> Product2/3
  Subtract/1 -> Product1/2
  Switch2/1 -> Add/1
  Product3/1 -> Add1/3
  Product1/1 -> Add1/1
  Add1/1 -> Limiter/2(in), Interval Test/1
  outMin/1 -> Limiter/3(min)
  outMax/1 -> Limiter/1(max)
  Switch1/1 -> Lcc_facLambdaPIDController/1
  initValue/1 -> Switch1/2
  Limiter/1(return) -> Switch1/1
  Constant1/1 -> Switch1/3

== system M160_lib/Functions/Lcc/Two-point-controller/EdgeFalling ==
  signal : Inport
  Detect Decrease : simulink/Logic and Bit Operations/Detect Decrease  vinit=0.0  InputProcessing=Inherited  OutDataTypeStr=boolean
  return : Outport
  wires:
  Detect Decrease/1 -> return/1
  signal/1 -> Detect Decrease/1

== system M160_lib/Functions/Lcc/Two-point-controller/EdgeFalling1 ==
  signal : Inport
  Detect Decrease : simulink/Logic and Bit Operations/Detect Decrease  vinit=0.0  InputProcessing=Inherited  OutDataTypeStr=boolean
  return : Outport
  wires:
  signal/1 -> Detect Decrease/1
  Detect Decrease/1 -> return/1

== system M160_lib/Functions/Lcc/Two-point-controller/EdgeRising ==
  signal : Inport
  Detect Increase : simulink/Logic and Bit Operations/Detect Increase  vinit=0.0  InputProcessing=Inherited  OutDataTypeStr=boolean
  return : Outport
  wires:
  Detect Increase/1 -> return/1
  signal/1 -> Detect Increase/1

== system M160_lib/Functions/Lcc/Two-point-controller/EdgeRising1 ==
  signal : Inport
  Detect Increase : simulink/Logic and Bit Operations/Detect Increase  vinit=0.0  InputProcessing=Inherited  OutDataTypeStr=boolean
  return : Outport
  wires:
  signal/1 -> Detect Increase/1
  Detect Increase/1 -> return/1

== system M160_lib/Functions/Lcc/Two-point-controller/Integrator ==
  initEnable : Inport
  enable : Inport  Port=2
  in : Inport  Port=3
  deltaT : Inport  Port=4
  mx : Inport  Port=5
  mn : Inport  Port=6
  initValue : Inport  Port=7
  Add : Sum
  MATLAB Function : MATLAB Function  TreatAsAtomicUnit=on
  MinMax : MinMax  Function=max  Inputs=2
  MinMax1 : MinMax  Inputs=2
  Product1 : Product  OutDataTypeStr=Inherit: Same as first input
  Unit Delay : UnitDelay  SampleTime=-1
  Unit Delay1 : UnitDelay  SampleTime=-1
  return : Outport
  wires:
  deltaT/1 -> Product1/2
  in/1 -> Product1/1
  Product1/1 -> Add/1
  Add/1 -> MinMax1/1
  mx/1 -> MinMax1/2
  MinMax1/1 -> MinMax/1
  mn/1 -> MinMax/2
  Unit Delay/1 -> Add/2
  MinMax/1 -> Unit Delay/1, MATLAB Function/4(in)
  MATLAB Function/1(out) -> Unit Delay1/1
  enable/1 -> MATLAB Function/3(enable)
  initValue/1 -> MATLAB Function/2(initValue)
  initEnable/1 -> MATLAB Function/1(initEnable)
  Unit Delay1/1 -> return/1

== system M160_lib/Functions/Opm/ErrorCheck/Counter ==
  in : Inport
  Add1 : Sum
  Constant1 : Constant  OutDataTypeStr=single
  Constant2 : Constant  Value=0  OutDataTypeStr=single
  MATLAB Function : MATLAB Function  TreatAsAtomicUnit=on
  Switch2 : Switch  Threshold=1
  Unit Delay1 : UnitDelay  SampleTime=-1
  Out1 : Outport
  wires:
  in/1 -> MATLAB Function/1(u)
  MATLAB Function/1(y) -> Switch2/2
  Add1/1 -> Unit Delay1/1, Switch2/1
  Constant2/1 -> Switch2/3
  Switch2/1 -> Out1/1
  Unit Delay1/1 -> Add1/2
  Constant1/1 -> Add1/1

== system M160_lib/Functions/Opm/ErrorCheck/Counter1 ==
  in : Inport
  Add1 : Sum
  Constant1 : Constant  OutDataTypeStr=single
  Constant2 : Constant  Value=0  OutDataTypeStr=single
  MATLAB Function : MATLAB Function  TreatAsAtomicUnit=on
  Switch2 : Switch  Threshold=1
  Unit Delay1 : UnitDelay  SampleTime=-1
  Out1 : Outport
  wires:
  Constant1/1 -> Add1/1
  Unit Delay1/1 -> Add1/2
  Switch2/1 -> Out1/1
  Constant2/1 -> Switch2/3
  Add1/1 -> Switch2/1, Unit Delay1/1
  MATLAB Function/1(y) -> Switch2/2
  in/1 -> MATLAB Function/1(u)

== system M160_lib/Functions/Opm/ErrorCheck/Counter2 ==
  in : Inport
  Add1 : Sum
  Constant1 : Constant  OutDataTypeStr=single
  Constant2 : Constant  Value=0  OutDataTypeStr=single
  MATLAB Function : MATLAB Function  TreatAsAtomicUnit=on
  Switch2 : Switch  Threshold=1
  Unit Delay1 : UnitDelay  SampleTime=-1
  Out1 : Outport
  wires:
  in/1 -> MATLAB Function/1(u)
  MATLAB Function/1(y) -> Switch2/2
  Add1/1 -> Unit Delay1/1, Switch2/1
  Constant2/1 -> Switch2/3
  Switch2/1 -> Out1/1
  Unit Delay1/1 -> Add1/2
  Constant1/1 -> Add1/1

== system M160_lib/Functions/Opm/OpMode/EdgeRising ==
  signal : Inport
  Detect Increase : simulink/Logic and Bit Operations/Detect Increase  vinit=0.0  InputProcessing=Inherited  OutDataTypeStr=boolean
  return : Outport
  wires:
  signal/1 -> Detect Increase/1
  Detect Increase/1 -> return/1

== system M160_lib/Functions/Opm/Opm_ErrorCheck/ECU_FcnCallTrigger_Source_DownStream ==
  ECU_FcnCallTrigger_Source_SFcn : S-Function  Tag=ECU_FcnCallTrigger_Source_SFcn  Description=Internal S-function for custom block ECU_FcnCallTrigger_Source. Do not rename!  FunctionName=ehooks_fcncalltrigger_source  Parameters=FunctionBlockId, FunctionCName, ProcessName, TaskPeriod, TaskPriority  EnableBusSupport=off  mask(ECU_FcnCallTrigger_Source_SFcn){FunctionCName=Opm_ErrorCheck, FunctionBlockId=SmartM160/Functions/Opm/Opm_ErrorCheck, ProcessName=BypEasyhooks_1ms_Pre_Proc, TaskPriority=0, TaskPeriod=1}
      mask prompts: FunctionCName "Function C name"; FunctionBlockId "Function block identifier"; ProcessName "Process name"; TaskPriority "Task priority (0..255)"; TaskPeriod "Sample time (0 for asynchronous operation)"
      mask help: Internal S-function for custom block ECU_FcnCallTrigger_Source. Do not rename!
      mask Display: disp('EHOOKS ECU Trigger\nSource S-Function')
  TriggerOut : Outport
  wires:
  ECU_FcnCallTrigger_Source_SFcn/1 -> TriggerOut/1

== system M160_lib/Functions/Opm/Opm_set/ECU_FcnCallTrigger_Source_DownStream ==
  ECU_FcnCallTrigger_Source_SFcn : S-Function  Tag=ECU_FcnCallTrigger_Source_SFcn  Description=Internal S-function for custom block ECU_FcnCallTrigger_Source. Do not rename!  FunctionName=ehooks_fcncalltrigger_source  Parameters=FunctionBlockId, FunctionCName, ProcessName, TaskPeriod, TaskPriority  EnableBusSupport=off  mask(ECU_FcnCallTrigger_Source_SFcn){FunctionCName=Opm_set, FunctionBlockId=SmartM160/Functions/Opm/Opm_set, ProcessName=BypEasyhooks_100ms_Pre_Proc, TaskPriority=0, TaskPeriod=100}
      mask prompts: FunctionCName "Function C name"; FunctionBlockId "Function block identifier"; ProcessName "Process name"; TaskPriority "Task priority (0..255)"; TaskPeriod "Sample time (0 for asynchronous operation)"
      mask help: Internal S-function for custom block ECU_FcnCallTrigger_Source. Do not rename!
      mask Display: disp('EHOOKS ECU Trigger\nSource S-Function')
  TriggerOut : Outport
  wires:
  ECU_FcnCallTrigger_Source_SFcn/1 -> TriggerOut/1

== system M160_lib/Functions/T2t/ThrottleValveControl/EdgeFalling ==
  signal : Inport
  Detect Decrease : simulink/Logic and Bit Operations/Detect Decrease  vinit=0.0  InputProcessing=Inherited  OutDataTypeStr=boolean
  return : Outport
  wires:
  Detect Decrease/1 -> return/1
  signal/1 -> Detect Decrease/1

== system M160_lib/Functions/T2t/ThrottleValveControl/PID_Limit_AWU ==
  Tn : Inport
  Tv : Inport  Port=2
  Ta : Inport  Port=3
  Kp : Inport  Port=4
  in : Inport  Port=5
  initValue : Inport  Port=6
  outMax : Inport  Port=7
  outMin : Inport  Port=8
  Add : Sum  OutDataTypeStr=Inherit: Same as first input
  Add1 : Sum  Inputs=+++  OutDataTypeStr=Inherit: Same as first input
  Constant1 : Constant  Value=0.0  OutDataTypeStr=single
  Constant10 : Constant  Value=0.0  OutDataTypeStr=single
  Divide : Product  Inputs=*/  OutDataTypeStr=Inherit: Same as first input
  Divide1 : Product  Inputs=*/  OutDataTypeStr=Inherit: Same as first input
  Interval Test : simulink/Logic and Bit Operations/Interval Test  IntervalClosedRight=on  uplimit=T2t_ThrValveReqCorrMax  IntervalClosedLeft=on  lowlimit=T2t_ThrValveReqCorrMin  OutDataTypeStr=boolean
  Limiter : Subsystem
      mask Description: Limiter
      mask Display: image(imread('Limiter.jpg'))
  Product : Product  OutDataTypeStr=Inherit: Same as first input
  Product1 : Product  OutDataTypeStr=Inherit: Same as first input
  Product2 : Product  Inputs=3  OutDataTypeStr=Inherit: Same as first input
  Product3 : Product  OutDataTypeStr=Inherit: Same as first input
  Subtract : Sum  Inputs=+-  OutDataTypeStr=Inherit: Same as first input
  Switch1 : Switch  Threshold=1
  Switch2 : Switch  Threshold=1
  Unit Delay1 : UnitDelay  SampleTime=-1
  Unit Delay2 : UnitDelay  SampleTime=-1
  Unit Delay3 : UnitDelay  SampleTime=-1
  T2t_facThrValveReqCorr : Outport
  wires:
  Constant10/1 -> Switch2/3
  Product2/1 -> Switch2/1
  Interval Test/1 -> Switch2/2
  Unit Delay2/1 -> Add/2, Add1/2
  Add/1 -> Unit Delay2/1
  Unit Delay1/1 -> Subtract/2
  Kp/1 -> Product/1, Product3/2, Divide1/1
  Tv/1 -> Product/2
  Product/1 -> Divide/1
  Ta/1 -> Product2/1, Divide/2
  Divide/1 -> Product1/1
  Tn/1 -> Divide1/2
  in/1 -> Product2/2, Product3/1, Subtract/1, Unit Delay1/1  "inOLD"
  Divide1/1 -> Product2/3
  Subtract/1 -> Product1/2
  Switch2/1 -> Add/1
  Product3/1 -> Add1/3
  Product1/1 -> Add1/1
  Add1/1 -> Limiter/2(in), Interval Test/1
  outMin/1 -> Limiter/3(min)
  outMax/1 -> Limiter/1(max)
  Switch1/1 -> T2t_facThrValveReqCorr/1
  Constant1/1 -> Switch1/1
  Limiter/1(return) -> Switch1/3
  initValue/1 -> Unit Delay3/1
  Unit Delay3/1 -> Switch1/2

== system M160_lib/Functions/T2t/WastegateControl/PID_Limit_AWU ==
  Tn : Inport
  Tv : Inport  Port=2
  Ta : Inport  Port=3
  Kp : Inport  Port=4
  in : Inport  Port=5
  initValue : Inport  Port=6
  outMax : Inport  Port=7
  outMin : Inport  Port=8
  Add : Sum  OutDataTypeStr=Inherit: Same as first input
  Add1 : Sum  Inputs=+++  OutDataTypeStr=Inherit: Same as first input
  Constant10 : Constant  Value=0.0  OutDataTypeStr=single
  Constant2 : Constant  Value=0.01  OutDataTypeStr=single
  Divide : Product  Inputs=*/  OutDataTypeStr=Inherit: Same as first input
  Divide1 : Product  Inputs=*/  OutDataTypeStr=Inherit: Same as first input
  Interval Test : simulink/Logic and Bit Operations/Interval Test  IntervalClosedRight=on  uplimit=1  IntervalClosedLeft=on  lowlimit=-1  OutDataTypeStr=boolean
  Limiter : Subsystem
      mask Description: Limiter
      mask Display: image(imread('Limiter.jpg'))
  Product : Product  OutDataTypeStr=Inherit: Same as first input
  Product1 : Product  OutDataTypeStr=Inherit: Same as first input
  Product2 : Product  Inputs=3  OutDataTypeStr=Inherit: Same as first input
  Product3 : Product  OutDataTypeStr=Inherit: Same as first input
  Subtract : Sum  Inputs=+-  OutDataTypeStr=Inherit: Same as first input
  Switch2 : Switch  Threshold=1
  Switch3 : Switch  Threshold=1
  Unit Delay1 : UnitDelay  SampleTime=-1
  Unit Delay2 : UnitDelay  SampleTime=-1
  T2t_facWastegateReqCorr : Outport
  wires:
  outMax/1 -> Limiter/1(max)
  outMin/1 -> Limiter/3(min)
  Add1/1 -> Interval Test/1, Limiter/2(in)
  Product1/1 -> Add1/1
  Product3/1 -> Add1/3
  Switch2/1 -> Add/1
  Subtract/1 -> Product1/2
  Divide1/1 -> Product2/3
  in/1 -> Unit Delay1/1, Subtract/1, Product3/1, Product2/2  "inOLD"
  Tn/1 -> Divide1/2
  Divide/1 -> Product1/1
  Ta/1 -> Divide/2, Product2/1
  Product/1 -> Divide/1
  Tv/1 -> Product/2
  Kp/1 -> Divide1/1, Product3/2, Product/1
  Unit Delay1/1 -> Subtract/2
  Add/1 -> Unit Delay2/1
  Unit Delay2/1 -> Add1/2, Add/2
  Interval Test/1 -> Switch2/2
  Product2/1 -> Switch2/1
  Constant10/1 -> Switch2/3
  Constant2/1 -> Switch3/3
  initValue/1 -> Switch3/2
  Switch3/1 -> T2t_facWastegateReqCorr/1
  Limiter/1(return) -> Switch3/1

== system M160_lib/Functions/Tqs/EngSpdControl/PID_Limit_AWU ==
  Tn : Inport
  Tv : Inport  Port=2
  Ta : Inport  Port=3
  Kp : Inport  Port=4
  in : Inport  Port=5
  initValue : Inport  Port=6
  outMax : Inport  Port=7
  outMin : Inport  Port=8
  Add : Sum  OutDataTypeStr=Inherit: Same as first input
  Add1 : Sum  Inputs=+++  OutDataTypeStr=Inherit: Same as first input
  Constant1 : Constant  Value=0.0  OutDataTypeStr=single
  Constant10 : Constant  Value=0.0  OutDataTypeStr=single
  Divide : Product  Inputs=*/  OutDataTypeStr=Inherit: Same as first input
  Divide1 : Product  Inputs=*/  OutDataTypeStr=Inherit: Same as first input
  Interval Test : simulink/Logic and Bit Operations/Interval Test  IntervalClosedRight=on  uplimit=Tqs_tqIdleSpdCtrlMax  IntervalClosedLeft=on  lowlimit=Tqs_tqIdleSpdCtrlMin  OutDataTypeStr=boolean
  Limiter : Subsystem
      mask Description: Limiter
      mask Display: image(imread('Limiter.jpg'))
  Product : Product  OutDataTypeStr=Inherit: Same as first input
  Product1 : Product  OutDataTypeStr=Inherit: Same as first input
  Product2 : Product  Inputs=3  OutDataTypeStr=Inherit: Same as first input
  Product3 : Product  OutDataTypeStr=Inherit: Same as first input
  Subtract : Sum  Inputs=+-  OutDataTypeStr=Inherit: Same as first input
  Switch1 : Switch  Threshold=1
  Switch2 : Switch  Threshold=1
  Unit Delay1 : UnitDelay  SampleTime=-1
  Unit Delay2 : UnitDelay  SampleTime=-1
  Tqs_tqIdleSpdCtrlCorr : Outport
  wires:
  Constant10/1 -> Switch2/3
  Product2/1 -> Switch2/1
  Interval Test/1 -> Switch2/2
  Unit Delay2/1 -> Add/2, Add1/2
  Add/1 -> Unit Delay2/1
  Unit Delay1/1 -> Subtract/2
  Kp/1 -> Product/1, Product3/2, Divide1/1
  Tv/1 -> Product/2
  Product/1 -> Divide/1
  Ta/1 -> Product2/1, Divide/2
  Divide/1 -> Product1/1
  Tn/1 -> Divide1/2
  in/1 -> Product2/2, Product3/1, Subtract/1, Unit Delay1/1  "inOLD"
  Divide1/1 -> Product2/3
  Subtract/1 -> Product1/2
  Switch2/1 -> Add/1
  Product3/1 -> Add1/3
  Product1/1 -> Add1/1
  Add1/1 -> Limiter/2(in), Interval Test/1
  outMin/1 -> Limiter/3(min)
  outMax/1 -> Limiter/1(max)
  Constant1/1 -> Switch1/3
  initValue/1 -> Switch1/2
  Switch1/1 -> Tqs_tqIdleSpdCtrlCorr/1
  Limiter/1(return) -> Switch1/1

== system M160_lib/Sensors/Cpc/Cpc_calc/Accumulator ==
  in : Inport
  initValue : Inport  Port=2
  Add : Sum
  MATLAB Function : MATLAB Function  TreatAsAtomicUnit=on
  Switch2 : Switch  Threshold=1
  Unit Delay : UnitDelay  SampleTime=-1
  Out2 : Outport
  wires:
  in/1 -> Add/1, MATLAB Function/1(u)
  Unit Delay/1 -> Add/2
  Switch2/1 -> Out2/1
  initValue/1 -> Switch2/3
  Add/1 -> Switch2/1, Unit Delay/1
  MATLAB Function/1(y) -> Switch2/2

== system M160_lib/Sensors/Cpc/Cpc_calc/Counter ==
  in : Inport
  Add1 : Sum
  Constant1 : Constant  OutDataTypeStr=single
  Constant2 : Constant  Value=0  OutDataTypeStr=single
  MATLAB Function : MATLAB Function  TreatAsAtomicUnit=on
  Switch2 : Switch  Threshold=1
  Unit Delay1 : UnitDelay  SampleTime=-1
  Out1 : Outport
  wires:
  Constant1/1 -> Add1/1
  Unit Delay1/1 -> Add1/2
  Switch2/1 -> Out1/1
  Constant2/1 -> Switch2/3
  Add1/1 -> Switch2/1, Unit Delay1/1
  MATLAB Function/1(y) -> Switch2/2
  in/1 -> MATLAB Function/1(u)
